simulink model "sim_rx160_two"  (R2020a)
settings: Solver=FixedStepAuto  StartTime=0.0  StopTime=25.0  FixedStep=0.0001  RelTol=1e-3
values from neighbouring files (symbols this model uses):
  cnc_comp = 1    [run_sim_two.m]
  ctc_switch = 0    [run_sim_two.m]
  ctrl_at_end = 1    [run_sim_two.m]
  ctrl_space = 1    [run_sim_two.m]
  ea_set = 4    [run_sim_two.m]
  ea_set2 = 4    [run_sim_two.m]
  ee_att_1 = 3    [run_sim_two.m]
  ee_att_2 = 4    [run_sim_two.m]
  f_des = [0;60;0;0;0;0]    [run_sim_two.m]
  force_ffwd = 1    [run_sim_two.m]
  fp = [p_ef;r_ef]    [run_sim_two.m]
  fp2 = [p_ef2;r_ef2]    [run_sim_two.m]
  frc_comp = 0    [run_sim_two.m]
  grv_comp = 1    [run_sim_two.m]
  ip = [p_ei;r_ei]    [run_sim_two.m]
  ip2 = [p_ei2;r_ei2]    [run_sim_two.m]
  K = 15000    [run_sim_two.m]
  Kc = 0.005    [run_sim_two.m]
  Kd = [10;10;10;7;7;7]    [run_sim_two.m]
  Kdf = [0;10;0;0;0;0]    [run_sim_two.m]
  Ki = [20;20;20;5;5;5]    [run_sim_two.m]
  Kif = [0;0.05;0;0;0;0]    [run_sim_two.m]
  Km = [1;1;1;1;1;1]    [run_sim_two.m]
  Kp = [2550;2250;2750;1150;850;650]    [run_sim_two.m]
  Kpf = [0;3;0;0;0;0]    [run_sim_two.m]
  orn_at_norm = 1    [run_sim_two.m]
  prdc_frc = 0    [run_sim_two.m]
  q_posIni = qi    [run_sim_two.m]
  robot_model_1 = 2    [run_sim_two.m]
  robot_model_2 = 3    [run_sim_two.m]
  rpt_num = 1    [run_sim_two.m]
  rpt_num2 = 10    [run_sim_two.m]
  Sf_diag = [0;1;0;0;0;0]    [run_sim_two.m]
  spr_comp = 1    [run_sim_two.m]
  switch_val = 30    [run_sim_two.m]
  Sx_diag = [1;0;1;1;1;1]    [run_sim_two.m]
  tf2 = rpt_num2 * period2    (= 30)    [run_sim_two.m]
  trj_profile = 3    [run_sim_two.m]
  trj_profile2 = 3    [run_sim_two.m]
  trj_space = 1    [run_sim_two.m]
  trj_space2 = 1    [run_sim_two.m]
  trj_type = 2    [run_sim_two.m]
  trj_type2 = 1    [run_sim_two.m]
undefined symbols (not defined in the file or in its folder): delta
libraries: simulink x2, vrlib x1
(part 4 of 4)

== matlab function sim_rx160_two/Robot 1 Control Algorithm/Base-to-End/spatialTrnsB2E1 ==
  data: q input; x input; a output; aB input
function a = sptTrnsAccB2E(q,x,aB)
    
    a = zeros(6,1);
    q_pos = q(1:6);
    q_vel = q(7:12);

    R_mat = [x(4:6) x(7:9) x(10:12)];
    R_dot = getR0_6dotMatrix(q_pos,q_vel);
    
    X_r_inv     = [R_mat' zeros(3,3);zeros(3,3) R_mat'];
    X_r_dot_inv = [R_dot' zeros(3,3);zeros(3,3) R_dot'];
    
    a = X_r_inv*aB + X_r_dot_inv*x(13:18);
    
end

== matlab function sim_rx160_two/Robot 1 Control Algorithm/Motion Controller/Proportional Gain ==
  data: Kp input; u input size=6; y output size=6
function y = fcn(Kp,u)

    sgn = zeros(6,1);
    
    sgn(1) = Kp(1)*u(1);
    sgn(2) = Kp(2)*u(2);
    sgn(3) = Kp(3)*u(3);
    sgn(4) = Kp(4)*u(4);
    sgn(5) = Kp(5)*u(5);
    sgn(6) = Kp(6)*u(6);

y = sgn;

== matlab function sim_rx160_two/Robot 1 Control Algorithm/Motion Controller/Inverse Mass Gain ==
  data: Km input; u input size=6; y output size=6
function y = fcn(Km,u)

    sgn = zeros(6,1);
    
    sgn(1) = u(1)/Km(1);
    sgn(2) = u(2)/Km(2);
    sgn(3) = u(3)/Km(3);
    sgn(4) = u(4)/Km(4);
    sgn(5) = u(5)/Km(5);
    sgn(6) = u(6)/Km(6);

y = sgn;

== matlab function sim_rx160_two/Robot 1 Control Algorithm/Force Controller/Inverse Mass Gain ==
  data: Km input; u input size=6; y output size=6
function y = fcn(Km,u)

    f = zeros(6,1);
    
    f(1) = u(1)/Km(1);
    f(2) = u(2)/Km(2);
    f(3) = u(3)/Km(3);
    f(4) = u(4)/Km(4);
    f(5) = u(5)/Km(5);
    f(6) = u(6)/Km(6);

y = f;

== matlab function sim_rx160_two/Robot 1 Control Algorithm/Base-to-End/spatialTrnsB2E2 ==
  data: x input; y output; v input
function y = sptTrnsTwistB2E(x,v)
    
    R_mat = [x(4:6) x(7:9) x(10:12)];
    
    X_r_inv = [R_mat' zeros(3,3);zeros(3,3) R_mat'];
    
    y = X_r_inv*v;
    
end

== matlab function sim_rx160_two/Robot 1 Control Algorithm/Base-to-End Wrench/spatialTrnsB2E ==
  data: x input; f_fbk input; f_fbkE output
function f_fbkE = sptTrnsWrnB2E(x,f_fbk)
    
    R_mat = [x(4:6) x(7:9) x(10:12)];
    
    X_r_inv = [R_mat' zeros(3,3);zeros(3,3) R_mat'];
    
    f_fbkE = X_r_inv*f_fbk;
        
end

== matlab function sim_rx160_two/Robot 1 Control Algorithm/Compliance/MATLAB Function ==
  data: y output; des input; Kc input; dXf input
function y = fcn(des,Kc,dXf)

    y = des;

    R_mat = [des(16:18) des(19:21) des(22:24)];
    R_new = R_mat*Rot_x(Kc*dXf(2));

    y(16:18) = R_new(1:3,1);
    y(19:21) = R_new(1:3,2);
    y(22:24) = R_new(1:3,3);
    
    function output = Rot_x(input)
        output = [	1	0           0
                    0	cos(input)  -sin(input)
                    0	sin(input)	cos(input)];
    end

%     function output = Rot_z(input)
%         output = [  cos(input)	-sin(input)	0	0
%                     sin(input)	 cos(input)	0	0
%                     0            0          1	0
%                     0            0          0	1 ];
%     end

end

== matlab function sim_rx160_two/Robot 1 Control Algorithm/Force Controller/ctrl switch ==
  data: switch_val input; ctrl_at_end input; y output size=1; f_fbk input
function y = fcn(switch_val,ctrl_at_end,f_fbk)

    if ctrl_at_end == 1
        fc_axis = 3;
    else
        fc_axis = 2;
    end
    
    if f_fbk(fc_axis) < switch_val
        y = 0;
    else
        y = 1;
    end
    
end

== matlab function sim_rx160_two/Environment/MATLAB Function3 ==
  data: x1 input; ee_att_1 input; x2 input size=18; K input; f_e output
function f_e = collisionModel(x1,ee_att_1,x2,K)

    L_srf = [0.64;0.64;0.00];
    
    T0_E_1 = eye(4);
    T0_E_1(1:3,1) = x1(4:6);
    T0_E_1(1:3,2) = x1(7:9);
    T0_E_1(1:3,3) = x1(10:12);
    T0_E_1(1:3,4) = x1(1:3);

    TI_0_1 = eye(4);
    TI_E_1 = TI_0_1*T0_E_1;
    
    TE_I_1 = eye(4);
    TE_I_1(1:3,1:3) = TI_E_1(1:3,1:3)';
    TE_I_1(1:3,4) = -TI_E_1(1:3,1:3)'*TI_E_1(1:3,4);
    
    T0_E_2 = eye(4);
    T0_E_2(1:3,1) = x2(4:6);
    T0_E_2(1:3,2) = x2(7:9);
    T0_E_2(1:3,3) = x2(10:12);
    T0_E_2(1:3,4) = x2(1:3);

    TI_0_2 = [  1,0,0,-0.28
                0,1,0, 2.43
                0,0,1, 0
                0,0,0, 1	];
            
    TI_E_2 = TI_0_2*T0_E_2;
    
    o_e1 = TI_E_1(1:3,4);
    o_e2 = TI_E_2(1:3,4);  
    z_e2 = TI_E_2(1:3,3);
    
    vert_srf_rel = [vertice_2d_gen(zeros(2,1),L_srf(1:2)),ones(4,1)]*TI_E_2'*TE_I_1';

    Mxy = [0,0];
    Axy = [vert_srf_rel(1,1),vert_srf_rel(1,2)];
    Bxy = [vert_srf_rel(2,1),vert_srf_rel(2,2)];
    Cxy = [vert_srf_rel(3,1),vert_srf_rel(3,2)];
    Dxy = [vert_srf_rel(4,1),vert_srf_rel(4,2)];

    coll_xy = pointInTriangle(Axy,Bxy,Cxy,Mxy) || pointInTriangle(Axy,Cxy,Dxy,Mxy);

    D = dot(z_e2,o_e2);

    d = (z_e2(1)*o_e1(1)+z_e2(2)*o_e1(2)+z_e2(3)*o_e1(3)-D)/sqrt(z_e2(1)^2+z_e2(2)^2+z_e2(3)^2);
    
    if ee_att_1 == 3
        if d < 0.0219
            K = 5014;
        end
    end
    
    coll_z = d < 0;
    
    if coll_xy && coll_z
        F = -K*abs(d)*z_e2;    
        f_e = [F(1);F(2);F(3);0;0;0];
    else
        f_e = zeros(6,1);
    end
    
    % floor
    if (o_e1(3) < -0.6)
        f_e(3) = K*(o_e1(3)-0.6);
    end
    
    function vert = vertice_2d_gen(O,L)

        vert = [O(1)-L(1)/2 O(2)-L(2)/2 0; ...
                O(1)-L(1)/2 O(2)+L(2)/2 0; ...
                O(1)+L(1)/2 O(2)+L(2)/2 0; ...
                O(1)+L(1)/2 O(2)-L(2)/2 0];

    end

    function out = pointInTriangle(P1,P2,P3,P)

        denom = ((P2(2) - P3(2))*(P1(1) - P3(1)) + (P3(1) - P2(1))*(P1(2) - P3(2)));

        a = ((P2(2) - P3(2))*(P(1) - P3(1)) + (P3(1) - P2(1))*(P(2) - P3(2))) / denom;
        b = ((P3(2) - P1(2))*(P(1) - P3(1)) + (P1(1) - P3(1))*(P(2) - P3(2))) / denom;
        c = 1 - a - b;

        out = 0 <= a && a <= 1 && 0 <= b && b <= 1 && 0 <= c && c <= 1;

    end

end

== matlab function sim_rx160_two/Robot 1 Control Algorithm/Motion Controller/Derivative Gain ==
  data: Kd input; u input size=6; y output size=6
function y = fcn(Kd,u)

    sgn = zeros(6,1);
    
    sgn(1) = Kd(1)*u(1);
    sgn(2) = Kd(2)*u(2);
    sgn(3) = Kd(3)*u(3);
    sgn(4) = Kd(4)*u(4);
    sgn(5) = Kd(5)*u(5);
    sgn(6) = Kd(6)*u(6);

y = sgn;

== matlab function sim_rx160_two/Robot 1 Control Algorithm/Motion Controller/Integral Gain ==
  data: Ki input; u input size=6; y output size=6
function y = fcn(Ki,u)

    sgn = zeros(6,1);
    
    sgn(1) = Ki(1)*u(1);
    sgn(2) = Ki(2)*u(2);
    sgn(3) = Ki(3)*u(3);
    sgn(4) = Ki(4)*u(4);
    sgn(5) = Ki(5)*u(5);
    sgn(6) = Ki(6)*u(6);

y = sgn;

== matlab function sim_rx160_two/Robot 1 Control Algorithm/Comp/Gravitational ==
  data: robot_model input; ee_att input; g input; q input size=6; tau_grv output size=6
function tau_grv = grvNE(robot_model,ee_att,g,q)

    [a_i,alpha_i,d_i,thetaPlus_i] = kinematicParametersOrigin(robot_model);

    d_e = getEElength(ee_att);

    [~,Th_i] = forwardGeometry(a_i,alpha_i,d_i,thetaPlus_i+q);

    Tn_E = [1 0 0 0
            0 1 0 0
            0 0 1 d_e
            0 0 0 1];

    Th_i(:,:,end) = Th_i(:,:,end)*Tn_E;
    
    Rh_i = zeros(3,3,6+1);
    Rh_i(:,:,1:6) = Th_i(1:3,1:3,:);

    %% Inverse Dynamics
    [m_i,ri_i_ci,Ii_i] = staticInertialParameters(robot_model,ee_att);

    rh_h_i = zeros(3,1,6+1); % +1 because of prcNE
    ci_i = zeros(3,1,6);
    for i1 = 1:6
        % origin i-1 to i on frame i-1
        rh_h_i(:,:,i1) = Th_i(1:3,4,i1);
        ci_i(:,:,i1) = m_i(i1) * ri_i_ci(:,:,i1);
    end
    
    p_obj.rh_h_i = rh_h_i;
    p_obj.ri_i_ci = ri_i_ci;
    p_obj.ci_i = ci_i;
    p_obj.Ii_i = Ii_i;
    p_obj.m_i = m_i;
    q_obj.Rh_i = Rh_i;

    tau_grv = prcNE(p_obj,q_obj,zeros(6,1),zeros(6,1),g);
    
end

== matlab function sim_rx160_two/Robot 1 Control Algorithm/Dyn Trns/MATLAB Function ==
  data: robot_model input; ee_att input; u input; tau output; q input
function tau = M_hat(robot_model,ee_att,u,q)

    tau = zeros(6,1);
    
    [a_i,alpha_i,d_i,thetaPlus_i] = kinematicParametersOrigin(robot_model);

    d_e = getEElength(ee_att);

    [~,Th_i] = forwardGeometry(a_i,alpha_i,d_i,thetaPlus_i+q);

    Tn_E = [1 0 0 0
            0 1 0 0
            0 0 1 d_e
            0 0 0 1];

    Th_i(:,:,end) = Th_i(:,:,end)*Tn_E;
    
    Rh_i = zeros(3,3,6+1);
    Rh_i(:,:,1:6) = Th_i(1:3,1:3,:);

    [m_i,ri_i_ci,Ii_i] = staticInertialParameters(robot_model,ee_att);

    rh_h_i = zeros(3,1,6+1); % +1 because of prcNE
    ci_i = zeros(3,1,6);
    for j = 1:6
        % origin i-1 to i on frame i-1
        rh_h_i(:,:,j) = Th_i(1:3,4,j);
        ci_i(:,:,j) = m_i(j) * ri_i_ci(:,:,j);
    end
    
    q_obj.Rh_i = Rh_i;
    p_obj.rh_h_i = rh_h_i;
    p_obj.m_i = m_i;
    p_obj.ci_i = ci_i;
    p_obj.Ii_i = Ii_i;

    v_hat = zeros(6,1);
    M_hat = zeros(6,6);
    for j = 1:6
        if j > 1
            v_hat(j-1) = 0;
        end
        v_hat(j) = 1;
        M_hat(j,:) = prcNE(p_obj,q_obj,zeros(6,1),v_hat,zeros(3,1));
    end
    
    tau = M_hat*u;

end
